simulink library "sensors_T2_lib"  (Simulink 6.6)
undefined symbols (not defined in the file or in its folder): alphavl_offset, alphavl_pos, alphavl_upwash, alphavr_offset, alphavr_pos, alphavr_upwash, betavl_offset, betavl_pos, betavl_sidewash, betavr_offset, betavr_pos, betavr_sidewash, POS_hi, POS_lo, Timestep
libraries: aeroutilslib x29, simulink_extras x6, SignalConditioning_lib x2, sensors_lib x1, simulink x1
(part 1 of 2)
settings Model: Creator=amurch  LastModifiedBy=amurch

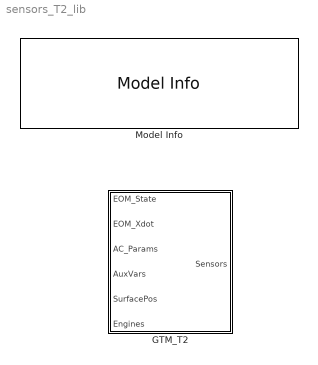
== system sensors_T2_lib ==
  GTM_T2 : Subsystem
      mask init:
      | if ~exist('MAG3TempComp','var')
      |     appendmws(Cal_params_T2)
      | end
  Model Info : simulink/Model-Wide Utilities/Model Info  SystemSampleTime=-1  InitialBlockCM=None  BlockCM=None  Frame=on  DisplayStringWithTags=|  HorizontalTextAlignment=Center  LeftAlignmentValue=0.5  SourceBlockDiagram=sensors_T2_lib  TagMaxNumber=20
      | GTM T2 Sensor Model Library
      | %<ModelVersion>
      | Las modified by %<LastModifiedBy> on %<LastModificationDate>

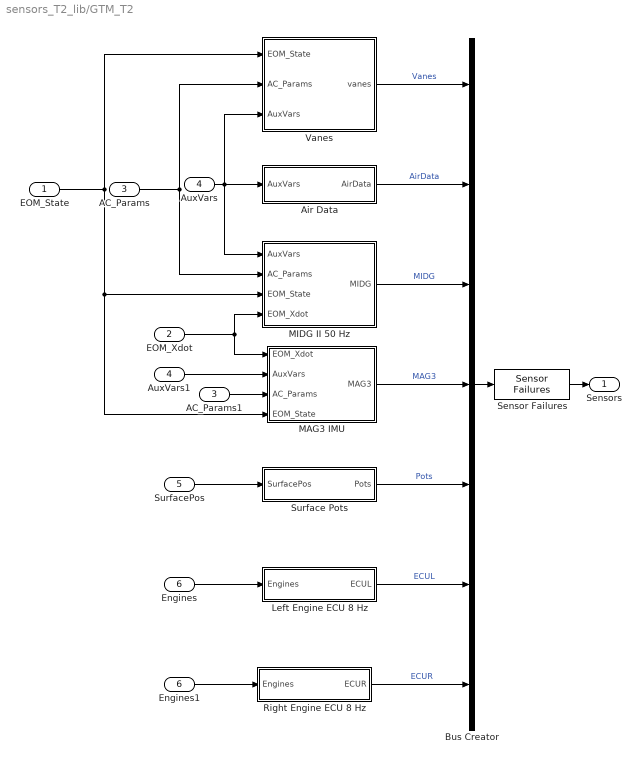
== system sensors_T2_lib/GTM_T2 ==
  EOM_State : Inport
  EOM_Xdot : Inport  Port=2
  AC_Params : Inport  Port=3
  AuxVars : Inport  Port=4
  SurfacePos : Inport  Port=5
  Engines : Inport  Port=6
  AC_Params1 : InportShadow  Port=3  LatchByCopyingInsideSignal=off
  Air Data : Subsystem
  AuxVars1 : InportShadow  Port=4  LatchByCopyingInsideSignal=off
  Bus Creator : BusCreator  Inputs=7
  Engines1 : InportShadow  Port=6  LatchByCopyingInsideSignal=off
  Left Engine ECU 8 Hz : Subsystem  SystemSampleTime=round(1/Timestep/8)*Timestep
  MAG3 IMU : Subsystem
  MIDG II 50 Hz : Subsystem  SystemSampleTime=round(1/Timestep/50)*Timestep
  Right Engine ECU 8 Hz : Subsystem  SystemSampleTime=round(1/Timestep/8)*Timestep
  Sensor Failures : sensors_lib/Sensor Failures  SystemSampleTime=-1
  Surface Pots : Subsystem
  Vanes : Subsystem
  Sensors : Outport
  wires:
  Sensor Failures/1 -> Sensors/1
  Engines1/1 -> Right Engine ECU 8 Hz/1(Engines)
  Right Engine ECU 8 Hz/1(ECUR) -> Bus Creator/7  "ECUR"
  Bus Creator/1 -> Sensor Failures/1
  Vanes/1(vanes) -> Bus Creator/1  "Vanes"
  Air Data/1(AirData) -> Bus Creator/2  "AirData"
  MIDG II 50 Hz/1(MIDG) -> Bus Creator/3  "MIDG"
  Surface Pots/1(Pots) -> Bus Creator/5  "Pots"
  Left Engine ECU 8 Hz/1(ECUL) -> Bus Creator/6  "ECUL"
  MAG3 IMU/1(MAG3) -> Bus Creator/4  "MAG3"
  Engines/1 -> Left Engine ECU 8 Hz/1(Engines)
  SurfacePos/1 -> Surface Pots/1(SurfacePos)
  AuxVars/1 -> Air Data/1(AuxVars), Vanes/3(AuxVars), MIDG II 50 Hz/1(AuxVars)
  AC_Params/1 -> Vanes/2(AC_Params), MIDG II 50 Hz/2(AC_Params)
  EOM_State/1 -> Vanes/1(EOM_State), MIDG II 50 Hz/3(EOM_State), MAG3 IMU/4(EOM_State)
  EOM_Xdot/1 -> MIDG II 50 Hz/4(EOM_Xdot), MAG3 IMU/1(EOM_Xdot)
  AuxVars1/1 -> MAG3 IMU/2(AuxVars)
  AC_Params1/1 -> MAG3 IMU/3(AC_Params)

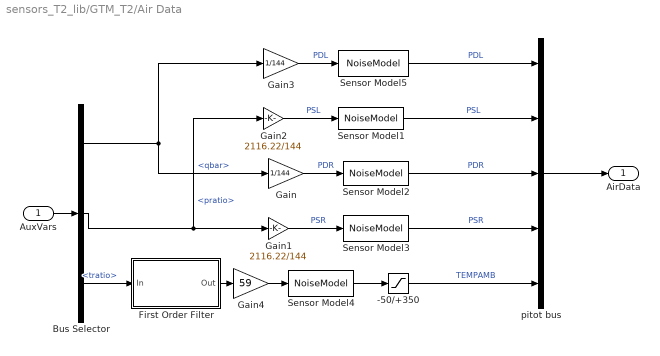
== system sensors_T2_lib/GTM_T2/Air Data ==
  AuxVars : Inport
  -50/+350 : Saturate  UpperLimit=350  LowerLimit=-50
  Bus Selector : BusSelector  OutputSignals=qbar,pratio,tratio
  First Order Filter : Subsystem  mask(first order filter){tau=6}
      mask help:
      | __1__
      |  tau s+1
      |
      | First order filter  transfer function
      | with integrator IC = input  at time=0
      | If tau < Simulation Timestep, input is passed through unchanged
      | Simulation timestep must be a variable in the model/base workspace named
      | "Timestep"
      mask Help:
      | This block models a first order filter with the initial condition
      | on the integrator set to the steady state value for constant input.
      | time constant is an input
      mask Display: fprintf('  1\n--------------\n %2.1g s + 1', tau)
  Gain : Gain  Gain=1/144
  Gain1 : Gain  Gain=2116.22/144
  Gain2 : Gain  Gain=2116.22/144
  Gain3 : Gain  Gain=1/144
  Gain4 : Gain  Gain=59
  Sensor Model1 : aeroutilslib/NoiseModel  SystemSampleTime=-1  noise_on=SensorNoise.On  sigma=SensorNoise.static_press.Std  seed=879234  bias=SensorNoise.static_press.Bias  scf=SensorNoise.static_press.Scf
  Sensor Model2 : aeroutilslib/NoiseModel  SystemSampleTime=-1  noise_on=SensorNoise.On  sigma=SensorNoise.dyn_press.Std  seed=848234  bias=SensorNoise.dyn_press.Bias  scf=SensorNoise.dyn_press.Scf
  Sensor Model3 : aeroutilslib/NoiseModel  SystemSampleTime=-1  noise_on=SensorNoise.On  sigma=SensorNoise.static_press.Std  seed=878634  bias=SensorNoise.static_press.Bias  scf=SensorNoise.static_press.Scf
  Sensor Model4 : aeroutilslib/NoiseModel  SystemSampleTime=-1  noise_on=SensorNoise.On  sigma=SensorNoise.tempamb.Std  seed=878634  bias=SensorNoise.tempamb.Bias  scf=SensorNoise.tempamb.Scf
  Sensor Model5 : aeroutilslib/NoiseModel  SystemSampleTime=-1  noise_on=SensorNoise.On  sigma=SensorNoise.dyn_press.Std  seed=878239  bias=SensorNoise.dyn_press.Bias  scf=SensorNoise.dyn_press.Scf
  pitot bus : BusCreator  Inputs=5
  AirData : Outport
  wires:
  AuxVars/1 -> Bus Selector/1
  pitot bus/1 -> AirData/1
  Bus Selector/1 -> Gain/1, Gain3/1  "<qbar>"
  Bus Selector/2 -> Gain1/1, Gain2/1  "<pratio>"
  Gain/1 -> Sensor Model2/1  "PDR"
  Gain1/1 -> Sensor Model3/1  "PSR"
  Gain3/1 -> Sensor Model5/1  "PDL"
  Gain2/1 -> Sensor Model1/1  "PSL"
  Sensor Model5/1 -> pitot bus/1  "PDL"
  Sensor Model1/1 -> pitot bus/2  "PSL"
  Sensor Model2/1 -> pitot bus/3  "PDR"
  Sensor Model3/1 -> pitot bus/4  "PSR"
  Bus Selector/3 -> First Order Filter/1(In)  "<tratio>"
  Gain4/1 -> Sensor Model4/1
  Sensor Model4/1 -> -50/+350/1
  -50/+350/1 -> pitot bus/5  "TEMPAMB"
  First Order Filter/1(Out) -> Gain4/1

== system sensors_T2_lib/GTM_T2/Left Engine ECU 8 Hz ==
  Engines : Inport
  0.025 V resolution : Quantizer  QuantizationInterval=0.025
  4.6 deg C resolution : Quantizer  QuantizationInterval=4.6
  500 RPM resolution : Quantizer  QuantizationInterval=500
  8 Hz : ZeroOrderHold  SampleTime=round(1/Timestep/8)*Timestep
  Bus Creator : BusCreator  Inputs=5
  Bus Selector : BusSelector  OutputSignals=RPML,EGTL,THROTLC,PUMPVL
  Gain : Gain
  Mode: 1 = on : Constant
  RT : RateTransition
  ECUL : Outport
  wires:
  Gain/1 -> Bus Creator/3  "ENGTL"
  Bus Selector/4 -> 0.025 V resolution/1  "<PUMPVL>"
  Bus Selector/2 -> 4.6 deg C resolution/1  "<EGTL>"
  8 Hz/1 -> RT/1
  Bus Creator/1 -> 8 Hz/1
  RT/1 -> ECUL/1
  Bus Selector/1 -> 500 RPM resolution/1  "<RPML>"
  500 RPM resolution/1 -> Bus Creator/1  "RPML"
  4.6 deg C resolution/1 -> Bus Creator/2  "EGTL"
  Bus Selector/3 -> Gain/1  "<THROTLC>"
  Mode: 1 = on/1 -> Bus Creator/5  "ENGML"
  0.025 V resolution/1 -> Bus Creator/4  "PUMPLV"
  Engines/1 -> Bus Selector/1

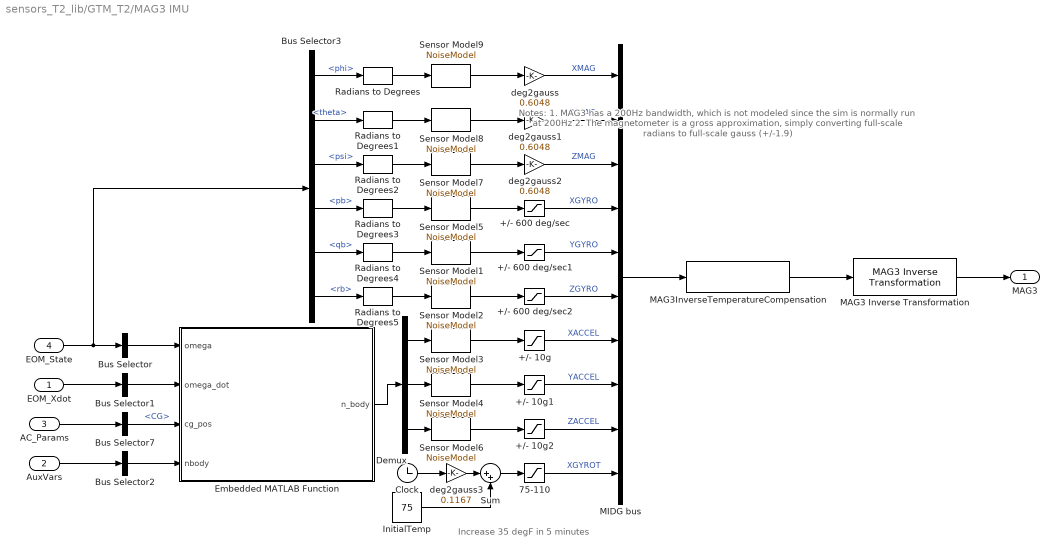
== system sensors_T2_lib/GTM_T2/MAG3 IMU ==
  note: Notes:
      |
      | 1. MAG3 has a 200Hz bandwidth, which is not modeled
      | since the sim is normally run at 200Hz
      |
      | 2.  The magnetometer is a gross approximation, simply converting
      | full-scale radians to full-scale gauss (+/-1.9)
  note: Increase 35 degF in 5 minutes
  EOM_Xdot : Inport
  AuxVars : Inport  Port=2
  AC_Params : Inport  Port=3
  EOM_State : Inport  Port=4
  +/- 10g : Saturate  UpperLimit=10  LowerLimit=-10
  +/- 10g1 : Saturate  UpperLimit=10  LowerLimit=-10
  +/- 10g2 : Saturate  UpperLimit=10  LowerLimit=-10
  +/- 600 deg/sec : Saturate  UpperLimit=600  LowerLimit=-600
  +/- 600 deg/sec1 : Saturate  UpperLimit=600  LowerLimit=-600
  +/- 600 deg/sec2 : Saturate  UpperLimit=600  LowerLimit=-600
  75-110 : Saturate  UpperLimit=110  LowerLimit=75
  Bus Selector : BusSelector  OutputSignals=pb,qb,rb  OutputAsBus=on
  Bus Selector1 : BusSelector  OutputSignals=pb_dot,qb_dot,rb_dot  OutputAsBus=on
  Bus Selector2 : BusSelector  OutputSignals=Ax,Ay,Az  OutputAsBus=on
  Bus Selector3 : BusSelector  OutputSignals=phi,theta,psi,pb,qb,rb
  Bus Selector7 : BusSelector  OutputSignals=CG
  Clock : Clock
      settings: Decimation=10
  Demux : Demux  Outputs=3
  Embedded MATLAB Function : Stateflow chart
  InitialTemp : Constant  Value=75
  MAG3 Inverse Transformation : SignalConditioning_lib/MAG3 Inverse Transformation  SystemSampleTime=-1
  MAG3InverseTemperatureCompensation : SignalConditioning_lib/MAG3InverseTemperatureCompensation  SystemSampleTime=-1
  MIDG bus : BusCreator  Inputs=10
  Radians to Degrees{,1..5} (6 alike) : simulink_extras/Transformations/Radians to Degrees  SystemSampleTime=-1
  Sensor Model1 : aeroutilslib/NoiseModel  SystemSampleTime=-1  noise_on=SensorNoise.On  sigma=SensorNoise.MAG3.qdeg.Std  seed=871234  bias=SensorNoise.MAG3.qdeg.Bias  scf=SensorNoise.MAG3.qdeg.Scf
  Sensor Model2 : aeroutilslib/NoiseModel  SystemSampleTime=-1  noise_on=SensorNoise.On  sigma=SensorNoise.MAG3.rdeg.Std  seed=878134  bias=SensorNoise.MAG3.rdeg.Bias  scf=SensorNoise.MAG3.rdeg.Scf
  Sensor Model3 : aeroutilslib/NoiseModel  SystemSampleTime=-1  noise_on=SensorNoise.On  sigma=SensorNoise.MAG3.nxbody.Std  seed=878234  bias=SensorNoise.MAG3.nxbody.Bias  scf=SensorNoise.MAG3.nxbody.Scf
  Sensor Model4 : aeroutilslib/NoiseModel  SystemSampleTime=-1  noise_on=SensorNoise.On  sigma=SensorNoise.MAG3.nybody.Std  seed=8782345  bias=SensorNoise.MAG3.nybody.Bias  scf=SensorNoise.MAG3.nybody.Scf
  Sensor Model5 : aeroutilslib/NoiseModel  SystemSampleTime=-1  noise_on=SensorNoise.On  sigma=SensorNoise.MAG3.pdeg.Std  seed=878233  bias=SensorNoise.MAG3.pdeg.Bias  scf=SensorNoise.MAG3.pdeg.Scf
  Sensor Model6 : aeroutilslib/NoiseModel  SystemSampleTime=-1  noise_on=SensorNoise.On  sigma=SensorNoise.MAG3.nzbody.Std  seed=878236  bias=SensorNoise.MAG3.nzbody.Bias  scf=SensorNoise.MAG3.nzbody.Scf
  Sensor Model7 : aeroutilslib/NoiseModel  SystemSampleTime=-1  noise_on=SensorNoise.On  sigma=SensorNoise.MAG3.psi.Std  seed=878232  bias=SensorNoise.MAG3.psi.Bias  scf=SensorNoise.MAG3.psi.Scf
  Sensor Model8 : aeroutilslib/NoiseModel  SystemSampleTime=-1  noise_on=SensorNoise.On  sigma=SensorNoise.MAG3.theta.Std  seed=878231  bias=SensorNoise.MAG3.theta.Bias  scf=SensorNoise.MAG3.theta.Scf
  Sensor Model9 : aeroutilslib/NoiseModel  SystemSampleTime=-1  noise_on=SensorNoise.On  sigma=SensorNoise.MAG3.phi.Std  seed=878230  bias=SensorNoise.MAG3.phi.Bias  scf=SensorNoise.MAG3.phi.Scf
  Sum : Sum  Inputs=|++
  deg2gauss : Gain  Gain=0.6048
  deg2gauss1 : Gain  Gain=0.6048
  deg2gauss2 : Gain  Gain=0.6048
  deg2gauss3 : Gain  Gain=0.1167
  MAG3 : Outport
  wires:
  75-110/1 -> MIDG bus/10  "XGYROT"
  Sum/1 -> 75-110/1
  deg2gauss3/1 -> Sum/1
  InitialTemp/1 -> Sum/2
  Clock/1 -> deg2gauss3/1
  MAG3 Inverse Transformation/1 -> MAG3/1
  MIDG bus/1 -> MAG3InverseTemperatureCompensation/1
  MAG3InverseTemperatureCompensation/1 -> MAG3 Inverse Transformation/1
  +/- 10g2/1 -> MIDG bus/9  "ZACCEL"
  +/- 10g1/1 -> MIDG bus/8  "YACCEL"
  +/- 10g/1 -> MIDG bus/7  "XACCEL"
  +/- 600 deg/sec2/1 -> MIDG bus/6  "ZGYRO"
  +/- 600 deg/sec1/1 -> MIDG bus/5  "YGYRO"
  +/- 600 deg/sec/1 -> MIDG bus/4  "XGYRO"
  deg2gauss2/1 -> MIDG bus/3  "ZMAG"
  deg2gauss1/1 -> MIDG bus/2  "YMAG"
  deg2gauss/1 -> MIDG bus/1  "XMAG"
  Sensor Model7/1 -> deg2gauss2/1
  Sensor Model8/1 -> deg2gauss1/1
  Sensor Model9/1 -> deg2gauss/1
  EOM_State/1 -> Bus Selector3/1, Bus Selector/1
  Embedded MATLAB Function/1(n_body) -> Demux/1
  Bus Selector/1 -> Embedded MATLAB Function/1(omega)
  EOM_Xdot/1 -> Bus Selector1/1
  Bus Selector3/1 -> Radians to Degrees/1  "<phi>"
  Bus Selector3/2 -> Radians to Degrees1/1  "<theta>"
  Bus Selector3/3 -> Radians to Degrees2/1  "<psi>"
  Bus Selector3/4 -> Radians to Degrees3/1  "<pb>"
  Bus Selector3/5 -> Radians to Degrees4/1  "<qb>"
  Bus Selector3/6 -> Radians to Degrees5/1  "<rb>"
  Demux/1 -> Sensor Model3/1
  Demux/2 -> Sensor Model4/1
  Demux/3 -> Sensor Model6/1
  Bus Selector1/1 -> Embedded MATLAB Function/2(omega_dot)
  Bus Selector7/1 -> Embedded MATLAB Function/3(cg_pos)  "<CG>"
  Radians to Degrees3/1 -> Sensor Model5/1
  Radians to Degrees4/1 -> Sensor Model1/1
  Radians to Degrees5/1 -> Sensor Model2/1
  Sensor Model1/1 -> +/- 600 deg/sec1/1
  Sensor Model2/1 -> +/- 600 deg/sec2/1
  Sensor Model3/1 -> +/- 10g/1
  Sensor Model4/1 -> +/- 10g1/1
  Sensor Model6/1 -> +/- 10g2/1
  Radians to Degrees/1 -> Sensor Model9/1
  Radians to Degrees1/1 -> Sensor Model8/1
  Radians to Degrees2/1 -> Sensor Model7/1
  Sensor Model5/1 -> +/- 600 deg/sec/1
  AC_Params/1 -> Bus Selector7/1
  AuxVars/1 -> Bus Selector2/1
  Bus Selector2/1 -> Embedded MATLAB Function/4(nbody)

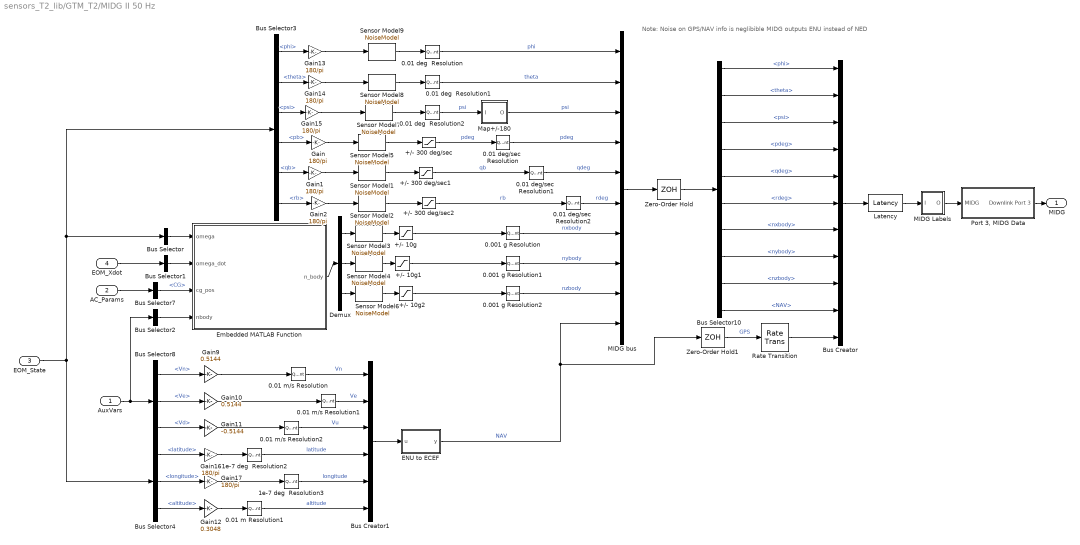
== system sensors_T2_lib/GTM_T2/MIDG II 50 Hz ==
  note: Note:  Noise on GPS/NAV info is neglibible
      | MIDG outputs ENU instead of NED
  AuxVars : Inport
  AC_Params : Inport  Port=2
  EOM_State : Inport  Port=3
  EOM_Xdot : Inport  Port=4
  +/- 10g : Saturate  UpperLimit=10  LowerLimit=-10
  +/- 10g1 : Saturate  UpperLimit=10  LowerLimit=-10
  +/- 10g2 : Saturate  UpperLimit=10  LowerLimit=-10
  +/- 300 deg/sec : Saturate  UpperLimit=300  LowerLimit=-300
  +/- 300 deg/sec1 : Saturate  UpperLimit=300  LowerLimit=-300
  +/- 300 deg/sec2 : Saturate  UpperLimit=300  LowerLimit=-300
  0.001 g Resolution : Quantizer  QuantizationInterval=0.001
  0.001 g Resolution1 : Quantizer  QuantizationInterval=0.001
  0.001 g Resolution2 : Quantizer  QuantizationInterval=0.001
  0.01 deg  Resolution : Quantizer  QuantizationInterval=0.01
  0.01 deg  Resolution1 : Quantizer  QuantizationInterval=0.01
  0.01 deg  Resolution2 : Quantizer  QuantizationInterval=0.01
  0.01 deg/sec  Resolution : Quantizer  QuantizationInterval=0.01
  0.01 deg/sec  Resolution1 : Quantizer  QuantizationInterval=0.01
  0.01 deg/sec  Resolution2 : Quantizer  QuantizationInterval=0.01
  0.01 m Resolution1 : Quantizer  QuantizationInterval=0.01
  0.01 m/s Resolution : Quantizer  QuantizationInterval=0.01
  0.01 m/s Resolution1 : Quantizer  QuantizationInterval=0.01
  0.01 m/s Resolution2 : Quantizer  QuantizationInterval=0.01
  1e-7 deg  Resolution2 : Quantizer  QuantizationInterval=1e-7
  1e-7 deg  Resolution3 : Quantizer  QuantizationInterval=1e-7
  Bus Creator : BusCreator  Inputs=11
  Bus Creator1 : BusCreator  Inputs=6
  Bus Selector : BusSelector  OutputSignals=pb,qb,rb  OutputAsBus=on
  Bus Selector1 : BusSelector  OutputSignals=pb_dot,qb_dot,rb_dot  OutputAsBus=on
  Bus Selector10 : BusSelector  OutputSignals=phi,theta,psi,pdeg,qdeg,rdeg,nxbody,nybody,nzbody,NAV
  Bus Selector2 : BusSelector  OutputSignals=Ax,Ay,Az  OutputAsBus=on
  Bus Selector3 : BusSelector  OutputSignals=phi,theta,psi,pb,qb,rb
  Bus Selector4 : BusSelector  OutputSignals=latitude,longitude,altitude
  Bus Selector7 : BusSelector  OutputSignals=CG
  Bus Selector8 : BusSelector  OutputSignals=Vn,Ve,Vd
  Demux : Demux  Outputs=3
  ENU to ECEF : Stateflow chart
  Embedded MATLAB Function : Stateflow chart
  Gain{,1..2,13..17} (8 alike) : Gain  Gain=180/pi
  Gain10 : Gain  Gain=0.5144
  Gain11 : Gain  Gain=-0.5144
  Gain12 : Gain  Gain=0.3048
  Gain9 : Gain  Gain=0.5144
  Latency : aeroutilslib/Latency  SystemSampleTime=-1  Latency=.04  timestep=Timestep
  MIDG Labels : Subsystem
  MIDG bus : BusCreator  Inputs=10
  Map+/-180 : Subsystem
  "Port 3, MIDG Data" : Subsystem
  Rate Transition : RateTransition  OutPortSampleTime=round(1/Timestep/50)*Timestep
  Sensor Model1 : aeroutilslib/NoiseModel  SystemSampleTime=-1  noise_on=SensorNoise.On  sigma=SensorNoise.MIDG.qdeg.Std  seed=871234  bias=SensorNoise.MIDG.qdeg.Bias  scf=SensorNoise.MIDG.qdeg.Scf
  Sensor Model2 : aeroutilslib/NoiseModel  SystemSampleTime=-1  noise_on=SensorNoise.On  sigma=SensorNoise.MIDG.rdeg.Std  seed=878134  bias=SensorNoise.MIDG.rdeg.Bias  scf=SensorNoise.MIDG.rdeg.Scf
  Sensor Model3 : aeroutilslib/NoiseModel  SystemSampleTime=-1  noise_on=SensorNoise.On  sigma=SensorNoise.MIDG.nxbody.Std  seed=878234  bias=SensorNoise.MIDG.nxbody.Bias  scf=SensorNoise.MIDG.nxbody.Scf
  Sensor Model4 : aeroutilslib/NoiseModel  SystemSampleTime=-1  noise_on=SensorNoise.On  sigma=SensorNoise.MIDG.nybody.Std  seed=8782345  bias=SensorNoise.MIDG.nybody.Bias  scf=SensorNoise.MIDG.nybody.Scf
  Sensor Model5 : aeroutilslib/NoiseModel  SystemSampleTime=-1  noise_on=SensorNoise.On  sigma=SensorNoise.MIDG.pdeg.Std  seed=878233  bias=SensorNoise.MIDG.pdeg.Bias  scf=SensorNoise.MIDG.pdeg.Scf
  Sensor Model6 : aeroutilslib/NoiseModel  SystemSampleTime=-1  noise_on=SensorNoise.On  sigma=SensorNoise.MIDG.nzbody.Std  seed=878236  bias=SensorNoise.MIDG.nzbody.Bias  scf=SensorNoise.MIDG.nzbody.Scf
  Sensor Model7 : aeroutilslib/NoiseModel  SystemSampleTime=-1  noise_on=SensorNoise.On  sigma=SensorNoise.MIDG.psi.Std  seed=878232  bias=SensorNoise.MIDG.psi.Bias  scf=SensorNoise.MIDG.psi.Scf
  Sensor Model8 : aeroutilslib/NoiseModel  SystemSampleTime=-1  noise_on=SensorNoise.On  sigma=SensorNoise.MIDG.theta.Std  seed=878231  bias=SensorNoise.MIDG.theta.Bias  scf=SensorNoise.MIDG.theta.Scf
  Sensor Model9 : aeroutilslib/NoiseModel  SystemSampleTime=-1  noise_on=SensorNoise.On  sigma=SensorNoise.MIDG.phi.Std  seed=878230  bias=SensorNoise.MIDG.phi.Bias  scf=SensorNoise.MIDG.phi.Scf
  Zero-Order Hold : ZeroOrderHold  SampleTime=round(1/Timestep/50)*Timestep
  Zero-Order Hold1 : ZeroOrderHold  SampleTime=round(1/Timestep/5)*Timestep
  MIDG : Outport
  wires:
  "Port 3, MIDG Data"/1(Downlink Port 3) -> MIDG/1
  Zero-Order Hold/1 -> Bus Selector10/1
  Rate Transition/1 -> Bus Creator/11
  Zero-Order Hold1/1 -> Rate Transition/1  "GPS"
  EOM_State/1 -> Bus Selector4/1, Bus Selector3/1, Bus Selector/1
  Embedded MATLAB Function/1(n_body) -> Demux/1
  EOM_Xdot/1 -> Bus Selector1/1
  Bus Selector3/1 -> Gain13/1  "<phi>"
  Bus Selector3/2 -> Gain14/1  "<theta>"
  Bus Selector3/3 -> Gain15/1  "<psi>"
  Bus Selector3/4 -> Gain/1  "<pb>"
  Bus Selector3/5 -> Gain1/1  "<qb>"
  Bus Selector3/6 -> Gain2/1  "<rb>"
  Demux/1 -> Sensor Model3/1
  Demux/2 -> Sensor Model4/1
  Demux/3 -> Sensor Model6/1
  Bus Selector7/1 -> Embedded MATLAB Function/3(cg_pos)  "<CG>"
  +/- 300 deg/sec/1 -> 0.01 deg/sec  Resolution/1  "pdeg"
  +/- 300 deg/sec1/1 -> 0.01 deg/sec  Resolution1/1  "qb"
  +/- 300 deg/sec2/1 -> 0.01 deg/sec  Resolution2/1  "rb"
  Gain/1 -> Sensor Model5/1
  Gain1/1 -> Sensor Model1/1
  Gain2/1 -> Sensor Model2/1
  +/- 10g/1 -> 0.001 g Resolution/1
  +/- 10g1/1 -> 0.001 g Resolution1/1
  Bus Creator1/1 -> ENU to ECEF/1(u)
  Bus Creator/1 -> Latency/1
  Sensor Model1/1 -> +/- 300 deg/sec1/1
  Sensor Model2/1 -> +/- 300 deg/sec2/1
  +/- 10g2/1 -> 0.001 g Resolution2/1
  Sensor Model3/1 -> +/- 10g/1
  Sensor Model4/1 -> +/- 10g1/1
  Sensor Model6/1 -> +/- 10g2/1
  Sensor Model7/1 -> 0.01 deg  Resolution2/1
  Sensor Model8/1 -> 0.01 deg  Resolution1/1
  Sensor Model9/1 -> 0.01 deg  Resolution/1
  0.01 deg  Resolution/1 -> MIDG bus/1  "phi"
  0.01 deg  Resolution1/1 -> MIDG bus/2  "theta"
  0.01 deg  Resolution2/1 -> Map+/-180/1(I)  "psi"
  1e-7 deg  Resolution2/1 -> Bus Creator1/4  "latitude"
  1e-7 deg  Resolution3/1 -> Bus Creator1/5  "longitude"
  0.001 g Resolution/1 -> MIDG bus/7  "nxbody"
  0.001 g Resolution1/1 -> MIDG bus/8  "nybody"
  0.001 g Resolution2/1 -> MIDG bus/9  "nzbody"
  0.01 m Resolution1/1 -> Bus Creator1/6  "altitude"
  Gain9/1 -> 0.01 m/s Resolution/1
  Gain10/1 -> 0.01 m/s Resolution1/1
  Gain11/1 -> 0.01 m/s Resolution2/1
  Gain12/1 -> 0.01 m Resolution1/1
  0.01 m/s Resolution/1 -> Bus Creator1/1  "Vn"
  0.01 m/s Resolution1/1 -> Bus Creator1/2  "Ve"
  0.01 m/s Resolution2/1 -> Bus Creator1/3  "Vu"
  0.01 deg/sec  Resolution1/1 -> MIDG bus/5  "qdeg"
  0.01 deg/sec  Resolution2/1 -> MIDG bus/6  "rdeg"
  MIDG bus/1 -> Zero-Order Hold/1
  Gain13/1 -> Sensor Model9/1
  Gain14/1 -> Sensor Model8/1
  Gain15/1 -> Sensor Model7/1
  Gain16/1 -> 1e-7 deg  Resolution2/1
  Gain17/1 -> 1e-7 deg  Resolution3/1
  AC_Params/1 -> Bus Selector7/1
  MIDG Labels/1(O) -> "Port 3, MIDG Data"/1(MIDG)
  Bus Selector10/1 -> Bus Creator/1  "<phi>"
  Bus Selector10/2 -> Bus Creator/2  "<theta>"
  Bus Selector10/3 -> Bus Creator/3  "<psi>"
  Bus Selector10/4 -> Bus Creator/4  "<pdeg>"
  Bus Selector10/5 -> Bus Creator/5  "<qdeg>"
  Bus Selector10/6 -> Bus Creator/6  "<rdeg>"
  Bus Selector10/7 -> Bus Creator/7  "<nxbody>"
  Bus Selector10/8 -> Bus Creator/8  "<nybody>"
  Bus Selector10/9 -> Bus Creator/9  "<nzbody>"
  Bus Selector10/10 -> Bus Creator/10  "<NAV>"
  Bus Selector8/1 -> Gain9/1  "<Vn>"
  Bus Selector8/2 -> Gain10/1  "<Ve>"
  Bus Selector8/3 -> Gain11/1  "<Vd>"
  Bus Selector4/1 -> Gain16/1  "<latitude>"
  Bus Selector4/2 -> Gain17/1  "<longitude>"
  Bus Selector4/3 -> Gain12/1  "<altitude>"
  ENU to ECEF/1(y) -> Zero-Order Hold1/1, MIDG bus/10  "NAV"
  AuxVars/1 -> Bus Selector8/1, Bus Selector2/1
  Sensor Model5/1 -> +/- 300 deg/sec/1
  0.01 deg/sec  Resolution/1 -> MIDG bus/4  "pdeg"
  Latency/1 -> MIDG Labels/1(I)
  Map+/-180/1(O) -> MIDG bus/3  "psi"
  Bus Selector/1 -> Embedded MATLAB Function/1(omega)
  Bus Selector1/1 -> Embedded MATLAB Function/2(omega_dot)
  Bus Selector2/1 -> Embedded MATLAB Function/4(nbody)

== system sensors_T2_lib/GTM_T2/Right Engine ECU 8 Hz ==
  Engines : Inport
  0.025 V resolution : Quantizer  QuantizationInterval=0.025
  4.6 deg C resolution : Quantizer  QuantizationInterval=4.6
  500 RPM resolution : Quantizer  QuantizationInterval=500
  8 Hz : ZeroOrderHold  SampleTime=round(1/Timestep/8)*Timestep
  Bus Creator : BusCreator  Inputs=5
  Bus Selector : BusSelector  OutputSignals=RPMR,EGTR,THROTRC,PUMPVR
  Gain : Gain
  Mode: 1 = on : Constant
  RT : RateTransition
  ECUR : Outport
  wires:
  Engines/1 -> Bus Selector/1
  0.025 V resolution/1 -> Bus Creator/4  "PUMPRV"
  Mode: 1 = on/1 -> Bus Creator/5  "ENGMR"
  Bus Selector/3 -> Gain/1  "<THROTRC>"
  4.6 deg C resolution/1 -> Bus Creator/2  "EGTR"
  500 RPM resolution/1 -> Bus Creator/1  "RPMR"
  Bus Selector/1 -> 500 RPM resolution/1  "<RPMR>"
  RT/1 -> ECUR/1
  Bus Creator/1 -> 8 Hz/1
  8 Hz/1 -> RT/1
  Bus Selector/2 -> 4.6 deg C resolution/1  "<EGTR>"
  Bus Selector/4 -> 0.025 V resolution/1  "<PUMPVR>"
  Gain/1 -> Bus Creator/3  "ENGTR"

== system sensors_T2_lib/GTM_T2/Surface Pots ==
  SurfacePos : Inport
  Bus Selector : BusSelector  OutputSignals=ELLOB,ELLIB,ELROB,ELRIB,AILL,AILR,RUDU,RUDL,FLAPLIB,FLAPLOB,FLAPRIB,FLAPROB  OutputAsBus=on
  Sensor Model5 : aeroutilslib/NoiseModel  SystemSampleTime=-1  noise_on=SensorNoise.On  sigma=SensorNoise.pots.Std  seed=878239  bias=SensorNoise.pots.Bias  scf=SensorNoise.pots.Scf
  Surface Labels : Subsystem
  Pots : Outport
  wires:
  Bus Selector/1 -> Sensor Model5/1
  SurfacePos/1 -> Bus Selector/1
  Sensor Model5/1 -> Surface Labels/1(I)
  Surface Labels/1(O) -> Pots/1

== system sensors_T2_lib/GTM_T2/Vanes ==
  EOM_State : Inport
  AC_Params : Inport  Port=2
  AuxVars : Inport  Port=3
  Bus Selector : BusSelector  OutputSignals=alpha,beta,tas
  Bus Selector1 : BusSelector  OutputSignals=pb,qb,rb  OutputAsBus=on
  Bus Selector2 : BusSelector  OutputSignals=CG
  Embedded MATLAB Function : Stateflow chart
  Sensor Model1 : aeroutilslib/NoiseModel  SystemSampleTime=-1  noise_on=SensorNoise.On  sigma=SensorNoise.beta.Std  seed=878224  bias=SensorNoise.beta.Bias  scf=SensorNoise.beta.Scf
  Sensor Model2 : aeroutilslib/NoiseModel  SystemSampleTime=-1  noise_on=SensorNoise.On  sigma=SensorNoise.alpha.Std  seed=878434  bias=SensorNoise.alpha.Bias  scf=SensorNoise.alpha.Scf
  Sensor Model3 : aeroutilslib/NoiseModel  SystemSampleTime=-1  noise_on=SensorNoise.On  sigma=SensorNoise.beta.Std  seed=878534  bias=SensorNoise.beta.Bias  scf=SensorNoise.beta.Scf
  Sensor Model5 : aeroutilslib/NoiseModel  SystemSampleTime=-1  noise_on=SensorNoise.On  sigma=SensorNoise.alpha.Std  seed=278234  bias=SensorNoise.alpha.Bias  scf=SensorNoise.alpha.Scf
  vane bus : BusCreator
  vanes : Outport
  wires:
  vane bus/1 -> vanes/1
  Embedded MATLAB Function/1(alphavl) -> Sensor Model5/1
  Embedded MATLAB Function/2(betavl) -> Sensor Model1/1
  Embedded MATLAB Function/3(alphavr) -> Sensor Model2/1
  Embedded MATLAB Function/4(betavr) -> Sensor Model3/1
  AuxVars/1 -> Bus Selector/1
  Bus Selector/1 -> Embedded MATLAB Function/2(alpha)  "<alpha>"
  Bus Selector/2 -> Embedded MATLAB Function/3(beta)  "<beta>"
  Bus Selector1/1 -> Embedded MATLAB Function/1(omega)
  EOM_State/1 -> Bus Selector1/1
  Bus Selector/3 -> Embedded MATLAB Function/4(vt)  "<tas>"
  AC_Params/1 -> Bus Selector2/1
  Bus Selector2/1 -> Embedded MATLAB Function/5(cg_pos)  "<CG>"
  Sensor Model5/1 -> vane bus/1  "ALPHAVL"
  Sensor Model1/1 -> vane bus/2  "BETAVL"
  Sensor Model2/1 -> vane bus/3  "ALPHAVR"
  Sensor Model3/1 -> vane bus/4  "BETAVR"

== system sensors_T2_lib/GTM_T2/Air Data/First Order Filter ==
  In : Inport
  Constant : Constant  Value=Timestep
  Constant1 : Constant  Value=tau
  Enabled Subsystem : Subsystem  TreatAsAtomicUnit=on
  Relational Operator : RelationalOperator  Operator=>  LogicOutDataTypeMode=Boolean
  Switch : Switch  Threshold=0.5
  Out : Outport
  wires:
  Constant1/1 -> Enabled Subsystem/2(tau), Relational Operator/1
  Enabled Subsystem/1(Out) -> Switch/1
  Switch/1 -> Out/1
  In/1 -> Enabled Subsystem/1(In), Switch/3
  Relational Operator/1 -> Enabled Subsystem/Enable, Switch/2
  Constant/1 -> Relational Operator/2

== system sensors_T2_lib/GTM_T2/MIDG II 50 Hz/MIDG Labels ==
  I : Inport
  Bus Creator : BusCreator  Inputs=33
  Demux : Demux  Outputs=33
  O : Outport
  wires:
  I/1 -> Demux/1
  Bus Creator/1 -> O/1
  Demux/2 -> Bus Creator/2  "theta"
  Demux/3 -> Bus Creator/3  "psi"
  Demux/4 -> Bus Creator/4  "pdeg"
  Demux/5 -> Bus Creator/5  "qdeg"
  Demux/6 -> Bus Creator/6  "rdeg"
  Demux/7 -> Bus Creator/7  "nxbody"
  Demux/8 -> Bus Creator/8  "nybody"
  Demux/9 -> Bus Creator/9  "nzbody"
  Demux/10 -> Bus Creator/10  "NAV_latitude"
  Demux/11 -> Bus Creator/11  "NAV_longitude"
  Demux/12 -> Bus Creator/12  "NAV_altitude"
  Demux/13 -> Bus Creator/13  "NAV_Vn"
  Demux/14 -> Bus Creator/14  "NAV_Ve"
  Demux/15 -> Bus Creator/15  "NAV_Vu"
  Demux/1 -> Bus Creator/1  "phi"
  Demux/16 -> Bus Creator/16  "NAV_XE"
  Demux/17 -> Bus Creator/17  "NAV_YE"
  Demux/18 -> Bus Creator/18  "NAV_ZE"
  Demux/19 -> Bus Creator/19  "NAV_VXE"
  Demux/20 -> Bus Creator/20  "NAV_VYE"
  Demux/21 -> Bus Creator/21  "NAV_VZE"
  Demux/22 -> Bus Creator/22  "GPS_latitude"
  Demux/23 -> Bus Creator/23  "GPS_longitude"
  Demux/24 -> Bus Creator/24  "GPS_altitude"
  Demux/25 -> Bus Creator/25  "GPS_Vn"
  Demux/26 -> Bus Creator/26  "GPS_Ve"
  Demux/27 -> Bus Creator/27  "GPS_Vu"
  Demux/28 -> Bus Creator/28  "GPS_XE"
  Demux/29 -> Bus Creator/29  "GPS_YE"
  Demux/30 -> Bus Creator/30  "GPS_ZE"
  Demux/31 -> Bus Creator/31  "GPS_VXE"
  Demux/32 -> Bus Creator/32  "GPS_VYE"
  Demux/33 -> Bus Creator/33  "GPS_VZE"

== system sensors_T2_lib/GTM_T2/MIDG II 50 Hz/Map+/-180 ==
  I : Inport
  Constant : Constant  Value=-360
  Constant1 : Constant  Value=0
  Sum : Sum  Inputs=|++
  if>180sub360 : Switch  Threshold=180
  O : Outport
  wires:
  if>180sub360/1 -> Sum/2
  Sum/1 -> O/1
  I/1 -> if>180sub360/2, Sum/1
  Constant1/1 -> if>180sub360/3
  Constant/1 -> if>180sub360/1

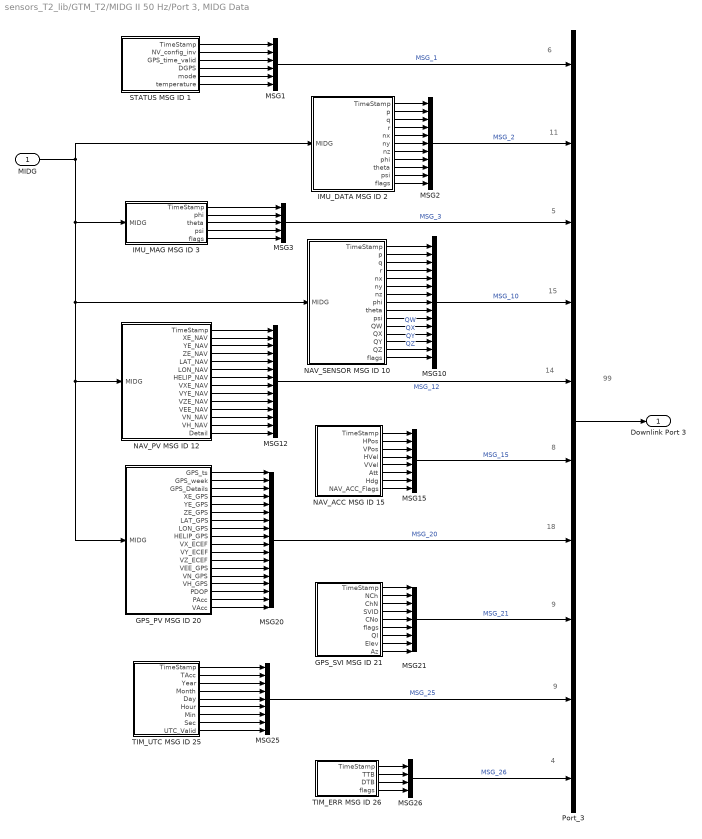
== system sensors_T2_lib/GTM_T2/MIDG II 50 Hz/Port 3, MIDG Data ==
  note: 99
  note: 4
  note: 9
  note: 9
  note: 18
  note: 8
  note: 14
  note: 15
  note: 5
  note: 11
  note: 6
  MIDG : Inport
  GPS_PV MSG ID 20 : Subsystem
  GPS_SVI MSG ID 21 : Subsystem
  IMU_DATA MSG ID 2 : Subsystem
  IMU_MAG MSG ID 3 : Subsystem
  MSG1 : BusCreator  Inputs=6
  MSG10 : BusCreator  Inputs=15
  MSG12 : BusCreator  Inputs=14
  MSG15 : BusCreator  Inputs=8
  MSG2 : BusCreator  Inputs=11
  MSG20 : BusCreator  Inputs=18
  MSG21 : BusCreator  Inputs=9
  MSG25 : BusCreator  Inputs=9
  MSG26 : BusCreator
  MSG3 : BusCreator  Inputs=5
  NAV_ACC MSG ID 15 : Subsystem
  NAV_PV MSG ID 12 : Subsystem
  NAV_SENSOR MSG ID 10 : Subsystem
  Port_3 : BusCreator  Inputs=10
  STATUS MSG ID 1 : Subsystem
  TIM_ERR MSG ID 26 : Subsystem
  TIM_UTC MSG ID 25 : Subsystem
  Downlink Port 3 : Outport
  wires:
  MIDG/1 -> IMU_DATA MSG ID 2/1(MIDG), NAV_SENSOR MSG ID 10/1(MIDG), GPS_PV MSG ID 20/1(MIDG), NAV_PV MSG ID 12/1(MIDG), IMU_MAG MSG ID 3/1(MIDG)
  Port_3/1 -> Downlink Port 3/1
  MSG21/1 -> Port_3/8  "MSG_21"
  MSG20/1 -> Port_3/7  "MSG_20"
  GPS_PV MSG ID 20/1(GPS_ts) -> MSG20/1
  GPS_PV MSG ID 20/2(GPS_week) -> MSG20/2
  GPS_PV MSG ID 20/3(GPS_Details) -> MSG20/3
  MSG10/1 -> Port_3/4  "MSG_10"
  MSG26/1 -> Port_3/10  "MSG_26"
  MSG25/1 -> Port_3/9  "MSG_25"
  MSG15/1 -> Port_3/6  "MSG_15"
  MSG12/1 -> Port_3/5  "MSG_12"
  MSG3/1 -> Port_3/3  "MSG_3"
  MSG2/1 -> Port_3/2  "MSG_2"
  MSG1/1 -> Port_3/1  "MSG_1"
  NAV_SENSOR MSG ID 10/15(flags) -> MSG10/15
  NAV_SENSOR MSG ID 10/14(QZ) -> MSG10/14  "QZ"
  NAV_SENSOR MSG ID 10/13(QY) -> MSG10/13  "QY"
  NAV_SENSOR MSG ID 10/12(QX) -> MSG10/12  "QX"
  NAV_SENSOR MSG ID 10/11(QW) -> MSG10/11  "QW"
  TIM_ERR MSG ID 26/4(flags) -> MSG26/4
  TIM_ERR MSG ID 26/3(DTB) -> MSG26/3
  TIM_ERR MSG ID 26/2(TTB) -> MSG26/2
  TIM_ERR MSG ID 26/1(TimeStamp) -> MSG26/1
  TIM_UTC MSG ID 25/9(UTC_Valid) -> MSG25/9
  TIM_UTC MSG ID 25/8(Sec) -> MSG25/8
  TIM_UTC MSG ID 25/7(Min) -> MSG25/7
  TIM_UTC MSG ID 25/6(Hour) -> MSG25/6
  TIM_UTC MSG ID 25/5(Day) -> MSG25/5
  TIM_UTC MSG ID 25/4(Month) -> MSG25/4
  TIM_UTC MSG ID 25/3(Year) -> MSG25/3
  TIM_UTC MSG ID 25/2(TAcc) -> MSG25/2
  TIM_UTC MSG ID 25/1(TimeStamp) -> MSG25/1
  GPS_SVI MSG ID 21/9(Az) -> MSG21/9
  GPS_SVI MSG ID 21/8(Elev) -> MSG21/8
  GPS_SVI MSG ID 21/7(QI) -> MSG21/7
  GPS_SVI MSG ID 21/6(flags) -> MSG21/6
  GPS_SVI MSG ID 21/5(CNo) -> MSG21/5
  GPS_SVI MSG ID 21/4(SVID) -> MSG21/4
  GPS_SVI MSG ID 21/3(ChN) -> MSG21/3
  GPS_SVI MSG ID 21/2(NCh) -> MSG21/2
  GPS_SVI MSG ID 21/1(TimeStamp) -> MSG21/1
  NAV_ACC MSG ID 15/8(NAV_ACC_Flags) -> MSG15/8
  NAV_ACC MSG ID 15/7(Hdg) -> MSG15/7
  NAV_ACC MSG ID 15/6(Att) -> MSG15/6
  NAV_ACC MSG ID 15/5(VVel) -> MSG15/5
  NAV_ACC MSG ID 15/4(HVel) -> MSG15/4
  NAV_ACC MSG ID 15/3(VPos) -> MSG15/3
  NAV_ACC MSG ID 15/2(HPos) -> MSG15/2
  NAV_ACC MSG ID 15/1(TimeStamp) -> MSG15/1
  NAV_SENSOR MSG ID 10/10(psi) -> MSG10/10
  NAV_SENSOR MSG ID 10/9(theta) -> MSG10/9
  NAV_SENSOR MSG ID 10/8(phi) -> MSG10/8
  NAV_SENSOR MSG ID 10/7(nz) -> MSG10/7
  NAV_SENSOR MSG ID 10/6(ny) -> MSG10/6
  NAV_SENSOR MSG ID 10/5(nx) -> MSG10/5
  NAV_SENSOR MSG ID 10/4(r) -> MSG10/4
  NAV_SENSOR MSG ID 10/3(q) -> MSG10/3
  NAV_SENSOR MSG ID 10/2(p) -> MSG10/2
  NAV_SENSOR MSG ID 10/1(TimeStamp) -> MSG10/1
  GPS_PV MSG ID 20/18(VAcc) -> MSG20/18
  GPS_PV MSG ID 20/17(PAcc) -> MSG20/17
  GPS_PV MSG ID 20/16(PDOP) -> MSG20/16
  GPS_PV MSG ID 20/15(VH_GPS) -> MSG20/15
  GPS_PV MSG ID 20/14(VN_GPS) -> MSG20/14
  GPS_PV MSG ID 20/13(VEE_GPS) -> MSG20/13
  GPS_PV MSG ID 20/12(VZ_ECEF) -> MSG20/12
  GPS_PV MSG ID 20/11(VY_ECEF) -> MSG20/11
  GPS_PV MSG ID 20/10(VX_ECEF) -> MSG20/10
  GPS_PV MSG ID 20/9(HELIP_GPS) -> MSG20/9
  GPS_PV MSG ID 20/8(LON_GPS) -> MSG20/8
  GPS_PV MSG ID 20/7(LAT_GPS) -> MSG20/7
  GPS_PV MSG ID 20/6(ZE_GPS) -> MSG20/6
  GPS_PV MSG ID 20/5(YE_GPS) -> MSG20/5
  GPS_PV MSG ID 20/4(XE_GPS) -> MSG20/4
  NAV_PV MSG ID 12/1(TimeStamp) -> MSG12/1
  NAV_PV MSG ID 12/2(XE_NAV) -> MSG12/2
  NAV_PV MSG ID 12/3(YE_NAV) -> MSG12/3
  NAV_PV MSG ID 12/4(ZE_NAV) -> MSG12/4
  NAV_PV MSG ID 12/5(LAT_NAV) -> MSG12/5
  NAV_PV MSG ID 12/6(LON_NAV) -> MSG12/6
  NAV_PV MSG ID 12/7(HELIP_NAV) -> MSG12/7
  NAV_PV MSG ID 12/8(VXE_NAV) -> MSG12/8
  NAV_PV MSG ID 12/9(VYE_NAV) -> MSG12/9
  NAV_PV MSG ID 12/10(VZE_NAV) -> MSG12/10
  NAV_PV MSG ID 12/11(VEE_NAV) -> MSG12/11
  NAV_PV MSG ID 12/12(VN_NAV) -> MSG12/12
  NAV_PV MSG ID 12/13(VH_NAV) -> MSG12/13
  NAV_PV MSG ID 12/14(Detail) -> MSG12/14
  IMU_MAG MSG ID 3/5(flags) -> MSG3/5
  IMU_MAG MSG ID 3/4(psi) -> MSG3/4
  IMU_MAG MSG ID 3/3(theta) -> MSG3/3
  IMU_MAG MSG ID 3/2(phi) -> MSG3/2
  IMU_MAG MSG ID 3/1(TimeStamp) -> MSG3/1
  IMU_DATA MSG ID 2/11(flags) -> MSG2/11
  IMU_DATA MSG ID 2/10(psi) -> MSG2/10
  IMU_DATA MSG ID 2/9(theta) -> MSG2/9
  IMU_DATA MSG ID 2/8(phi) -> MSG2/8
  IMU_DATA MSG ID 2/7(nz) -> MSG2/7
  IMU_DATA MSG ID 2/5(nx) -> MSG2/5
  IMU_DATA MSG ID 2/4(r) -> MSG2/4
  IMU_DATA MSG ID 2/3(q) -> MSG2/3
  IMU_DATA MSG ID 2/2(p) -> MSG2/2
  IMU_DATA MSG ID 2/1(TimeStamp) -> MSG2/1
  IMU_DATA MSG ID 2/6(ny) -> MSG2/6
  STATUS MSG ID 1/6(temperature) -> MSG1/6
  STATUS MSG ID 1/5(mode) -> MSG1/5
  STATUS MSG ID 1/4(DGPS) -> MSG1/4
  STATUS MSG ID 1/3(GPS_time_valid) -> MSG1/3
  STATUS MSG ID 1/2(NV_config_inv) -> MSG1/2
  STATUS MSG ID 1/1(TimeStamp) -> MSG1/1

== system sensors_T2_lib/GTM_T2/Surface Pots/Surface Labels ==
  I : Inport
  Bus Creator : BusCreator  Inputs=12
  Demux : Demux  Outputs=12
  O : Outport
  wires:
  Bus Creator/1 -> O/1
  Demux/12 -> Bus Creator/12  "FLAPROB"
  Demux/11 -> Bus Creator/11  "FLAPRIB"
  Demux/10 -> Bus Creator/10  "FLAPLOB"
  Demux/9 -> Bus Creator/9  "FLAPLIB"
  Demux/8 -> Bus Creator/8  "RUDL"
  Demux/7 -> Bus Creator/7  "RUDU"
  Demux/6 -> Bus Creator/6  "AILR"
  Demux/5 -> Bus Creator/5  "AILL"
  Demux/4 -> Bus Creator/4  "ELRIB"
  Demux/3 -> Bus Creator/3  "ELROB"
  Demux/2 -> Bus Creator/2  "ELLIB"
  Demux/1 -> Bus Creator/1  "ELLOB"
  I/1 -> Demux/1

== system sensors_T2_lib/GTM_T2/Air Data/First Order Filter/Enabled Subsystem ==
  In : Inport
  tau : Inport  Port=2
  Enable : EnablePort
  Divide : Product  Inputs=*/  OutScaling=2^-10
  Integrator : Integrator  InitialConditionSource=external  UpperSaturationLimit=POS_hi  LowerSaturationLimit=POS_lo
  Sum : Sum  Inputs=-+|  SaturateOnIntegerOverflow=on  InputSameDT=on
  Out : Outport
  wires:
  Sum/1 -> Divide/1  "Error"
  In/1 -> Sum/2, Integrator/2
  Integrator/1 -> Out/1, Sum/1  "Y"
  tau/1 -> Divide/2
  Divide/1 -> Integrator/1  "Ydot"

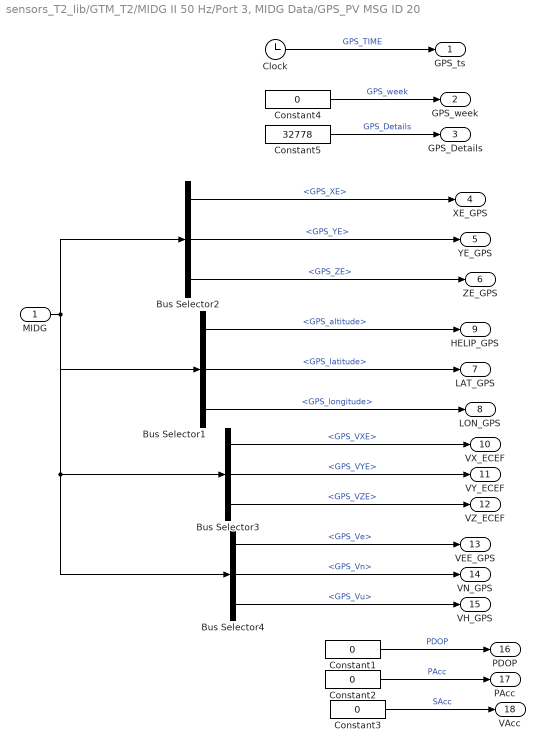
== system sensors_T2_lib/GTM_T2/MIDG II 50 Hz/Port 3, MIDG Data/GPS_PV MSG ID 20 ==
  MIDG : Inport
  Bus Selector1 : BusSelector  OutputSignals=GPS_altitude,GPS_latitude,GPS_longitude
  Bus Selector2 : BusSelector  OutputSignals=GPS_XE,GPS_YE,GPS_ZE
  Bus Selector3 : BusSelector  OutputSignals=GPS_VXE,GPS_VYE,GPS_VZE
  Bus Selector4 : BusSelector  OutputSignals=GPS_Ve,GPS_Vn,GPS_Vu
  Clock : Clock
      settings: Decimation=10
  Constant{1..4} (4 alike) : Constant  Value=0
  Constant5 : Constant  Value=32778
  GPS_ts : Outport
  GPS_week : Outport  Port=2
  GPS_Details : Outport  Port=3
  XE_GPS : Outport  Port=4
  YE_GPS : Outport  Port=5
  ZE_GPS : Outport  Port=6
  LAT_GPS : Outport  Port=7
  LON_GPS : Outport  Port=8
  HELIP_GPS : Outport  Port=9
  VX_ECEF : Outport  Port=10
  VY_ECEF : Outport  Port=11
  VZ_ECEF : Outport  Port=12
  VEE_GPS : Outport  Port=13
  VN_GPS : Outport  Port=14
  VH_GPS : Outport  Port=15
  PDOP : Outport  Port=16
  PAcc : Outport  Port=17
  VAcc : Outport  Port=18
  wires:
  Bus Selector2/3 -> ZE_GPS/1  "<GPS_ZE>"
  Bus Selector2/2 -> YE_GPS/1  "<GPS_YE>"
  Bus Selector2/1 -> XE_GPS/1  "<GPS_XE>"
  Bus Selector3/3 -> VZ_ECEF/1  "<GPS_VZE>"
  Bus Selector3/2 -> VY_ECEF/1  "<GPS_VYE>"
  Bus Selector3/1 -> VX_ECEF/1  "<GPS_VXE>"
  Constant5/1 -> GPS_Details/1  "GPS_Details"
  Constant4/1 -> GPS_week/1  "GPS_week"
  Clock/1 -> GPS_ts/1  "GPS_TIME"
  Constant3/1 -> VAcc/1  "SAcc"
  Constant2/1 -> PAcc/1  "PAcc"
  Constant1/1 -> PDOP/1  "PDOP"
  Bus Selector4/3 -> VH_GPS/1  "<GPS_Vu>"
  Bus Selector4/2 -> VN_GPS/1  "<GPS_Vn>"
  Bus Selector4/1 -> VEE_GPS/1  "<GPS_Ve>"
  Bus Selector1/3 -> LON_GPS/1  "<GPS_longitude>"
  Bus Selector1/2 -> LAT_GPS/1  "<GPS_latitude>"
  Bus Selector1/1 -> HELIP_GPS/1  "<GPS_altitude>"
  MIDG/1 -> Bus Selector2/1, Bus Selector4/1, Bus Selector3/1, Bus Selector1/1

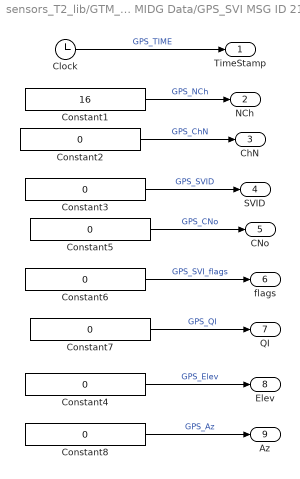
== system sensors_T2_lib/GTM_T2/MIDG II 50 Hz/Port 3, MIDG Data/GPS_SVI MSG ID 21 ==
  Clock : Clock
      settings: Decimation=10
  Constant1 : Constant  Value=16
  Constant{2..8} (7 alike) : Constant  Value=0
  TimeStamp : Outport
  NCh : Outport  Port=2
  ChN : Outport  Port=3
  SVID : Outport  Port=4
  CNo : Outport  Port=5
  flags : Outport  Port=6
  QI : Outport  Port=7
  Elev : Outport  Port=8
  Az : Outport  Port=9
  wires:
  Constant8/1 -> Az/1  "GPS_Az"
  Constant7/1 -> QI/1  "GPS_QI"
  Constant6/1 -> flags/1  "GPS_SVI_flags"
  Constant5/1 -> CNo/1  "GPS_CNo"
  Constant3/1 -> SVID/1  "GPS_SVID"
  Constant2/1 -> ChN/1  "GPS_ChN"
  Constant1/1 -> NCh/1  "GPS_NCh"
  Constant4/1 -> Elev/1  "GPS_Elev"
  Clock/1 -> TimeStamp/1  "GPS_TIME"

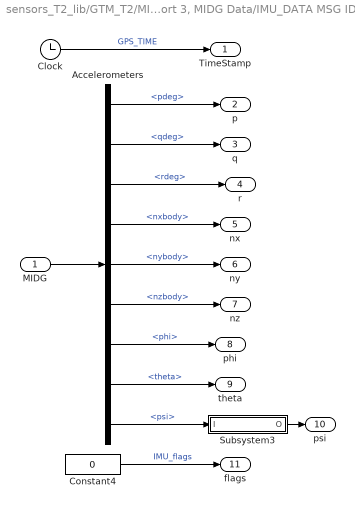
== system sensors_T2_lib/GTM_T2/MIDG II 50 Hz/Port 3, MIDG Data/IMU_DATA MSG ID 2 ==
  MIDG : Inport
  Accelerometers : BusSelector  OutputSignals=pdeg,qdeg,rdeg,nxbody,nybody,nzbody,phi,theta,psi
  Clock : Clock
      settings: Decimation=10
  Constant4 : Constant  Value=0
  Subsystem3 : Subsystem
      mask Display: disp('no windup 180')
  TimeStamp : Outport
  p : Outport  Port=2
  q : Outport  Port=3
  r : Outport  Port=4
  nx : Outport  Port=5
  ny : Outport  Port=6
  nz : Outport  Port=7
  phi : Outport  Port=8
  theta : Outport  Port=9
  psi : Outport  Port=10
  flags : Outport  Port=11
  wires:
  Accelerometers/9 -> Subsystem3/1(I)  "<psi>"
  Accelerometers/8 -> theta/1  "<theta>"
  Accelerometers/7 -> phi/1  "<phi>"
  Accelerometers/3 -> r/1  "<rdeg>"
  Accelerometers/2 -> q/1  "<qdeg>"
  Accelerometers/1 -> p/1  "<pdeg>"
  Subsystem3/1(O) -> psi/1
  Constant4/1 -> flags/1  "IMU_flags"
  Clock/1 -> TimeStamp/1  "GPS_TIME"
  Accelerometers/4 -> nx/1  "<nxbody>"
  Accelerometers/5 -> ny/1  "<nybody>"
  Accelerometers/6 -> nz/1  "<nzbody>"
  MIDG/1 -> Accelerometers/1

== system sensors_T2_lib/GTM_T2/MIDG II 50 Hz/Port 3, MIDG Data/IMU_MAG MSG ID 3 ==
  MIDG : Inport
  Clock : Clock
      settings: Decimation=10
  Constant4 : Constant  Value=0
  Magnetometer : BusSelector  OutputSignals=phi,theta,psi
  Subsystem3 : Subsystem
      mask Display: disp('no windup 180')
  TimeStamp : Outport
  phi : Outport  Port=2
  theta : Outport  Port=3
  psi : Outport  Port=4
  flags : Outport  Port=5
  wires:
  Subsystem3/1(O) -> psi/1
  Constant4/1 -> flags/1  "MAG_flags"
  Clock/1 -> TimeStamp/1  "GPS_TIME"
  Magnetometer/1 -> phi/1  "<phi>"
  Magnetometer/2 -> theta/1  "<theta>"
  Magnetometer/3 -> Subsystem3/1(I)  "<psi>"
  MIDG/1 -> Magnetometer/1

== system sensors_T2_lib/GTM_T2/MIDG II 50 Hz/Port 3, MIDG Data/NAV_ACC MSG ID 15 ==
  Clock : Clock
      settings: Decimation=10
  Constant{1..7} (7 alike) : Constant  Value=0
  TimeStamp : Outport
  HPos : Outport  Port=2
  VPos : Outport  Port=3
  HVel : Outport  Port=4
  VVel : Outport  Port=5
  Att : Outport  Port=6
  Hdg : Outport  Port=7
  NAV_ACC_Flags : Outport  Port=8
  wires:
  Constant7/1 -> Hdg/1  "Hdg"
  Constant6/1 -> Att/1  "Att"
  Constant5/1 -> VVel/1  "VVel"
  Constant3/1 -> HVel/1  "HVel"
  Constant2/1 -> VPos/1  "VPos"
  Constant1/1 -> HPos/1  "HPos"
  Constant4/1 -> NAV_ACC_Flags/1  "NAV_ACC_Flags"
  Clock/1 -> TimeStamp/1  "GPS_TIME"

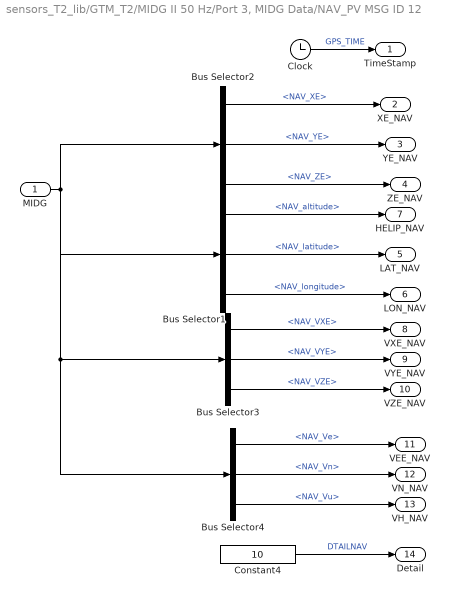
== system sensors_T2_lib/GTM_T2/MIDG II 50 Hz/Port 3, MIDG Data/NAV_PV MSG ID 12 ==
  MIDG : Inport
  Bus Selector1 : BusSelector  OutputSignals=NAV_altitude,NAV_latitude,NAV_longitude
  Bus Selector2 : BusSelector  OutputSignals=NAV_XE,NAV_YE,NAV_ZE
  Bus Selector3 : BusSelector  OutputSignals=NAV_VXE,NAV_VYE,NAV_VZE
  Bus Selector4 : BusSelector  OutputSignals=NAV_Ve,NAV_Vn,NAV_Vu
  Clock : Clock
      settings: Decimation=10
  Constant4 : Constant  Value=10
  TimeStamp : Outport
  XE_NAV : Outport  Port=2
  YE_NAV : Outport  Port=3
  ZE_NAV : Outport  Port=4
  LAT_NAV : Outport  Port=5
  LON_NAV : Outport  Port=6
  HELIP_NAV : Outport  Port=7
  VXE_NAV : Outport  Port=8
  VYE_NAV : Outport  Port=9
  VZE_NAV : Outport  Port=10
  VEE_NAV : Outport  Port=11
  VN_NAV : Outport  Port=12
  VH_NAV : Outport  Port=13
  Detail : Outport  Port=14
  wires:
  Bus Selector2/3 -> ZE_NAV/1  "<NAV_ZE>"
  Bus Selector2/2 -> YE_NAV/1  "<NAV_YE>"
  Bus Selector2/1 -> XE_NAV/1  "<NAV_XE>"
  Bus Selector3/3 -> VZE_NAV/1  "<NAV_VZE>"
  Bus Selector3/2 -> VYE_NAV/1  "<NAV_VYE>"
  Bus Selector3/1 -> VXE_NAV/1  "<NAV_VXE>"
  Constant4/1 -> Detail/1  "DTAILNAV"
  Clock/1 -> TimeStamp/1  "GPS_TIME"
  Bus Selector4/3 -> VH_NAV/1  "<NAV_Vu>"
  Bus Selector4/2 -> VN_NAV/1  "<NAV_Vn>"
  Bus Selector4/1 -> VEE_NAV/1  "<NAV_Ve>"
  Bus Selector1/3 -> LON_NAV/1  "<NAV_longitude>"
  Bus Selector1/2 -> LAT_NAV/1  "<NAV_latitude>"
  Bus Selector1/1 -> HELIP_NAV/1  "<NAV_altitude>"
  MIDG/1 -> Bus Selector2/1, Bus Selector4/1, Bus Selector3/1, Bus Selector1/1

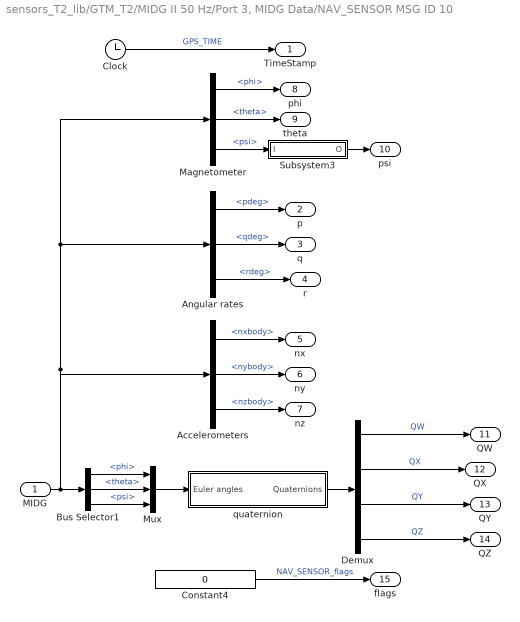
== system sensors_T2_lib/GTM_T2/MIDG II 50 Hz/Port 3, MIDG Data/NAV_SENSOR MSG ID 10 ==
  MIDG : Inport
  Accelerometers : BusSelector  OutputSignals=nxbody,nybody,nzbody
  Angular rates : BusSelector  OutputSignals=pdeg,qdeg,rdeg
  Bus Selector1 : BusSelector  OutputSignals=phi,theta,psi
  Clock : Clock
      settings: Decimation=10
  Constant4 : Constant  Value=0
  Demux : Demux
  Magnetometer : BusSelector  OutputSignals=phi,theta,psi
  Mux : Mux  Inputs=3
  Subsystem3 : Subsystem
      mask Display: disp('360 to +/-180')
  quaternion : Subsystem
  TimeStamp : Outport
  p : Outport  Port=2
  q : Outport  Port=3
  r : Outport  Port=4
  nx : Outport  Port=5
  ny : Outport  Port=6
  nz : Outport  Port=7
  phi : Outport  Port=8
  theta : Outport  Port=9
  psi : Outport  Port=10
  QW : Outport  Port=11
  QX : Outport  Port=12
  QY : Outport  Port=13
  QZ : Outport  Port=14
  flags : Outport  Port=15
  wires:
  Subsystem3/1(O) -> psi/1
  Constant4/1 -> flags/1  "NAV_SENSOR_flags"
  Clock/1 -> TimeStamp/1  "GPS_TIME"
  Angular rates/1 -> p/1  "<pdeg>"
  Angular rates/2 -> q/1  "<qdeg>"
  Angular rates/3 -> r/1  "<rdeg>"
  Accelerometers/1 -> nx/1  "<nxbody>"
  Accelerometers/2 -> ny/1  "<nybody>"
  Accelerometers/3 -> nz/1  "<nzbody>"
  Magnetometer/1 -> phi/1  "<phi>"
  Magnetometer/2 -> theta/1  "<theta>"
  Magnetometer/3 -> Subsystem3/1(I)  "<psi>"
  Bus Selector1/1 -> Mux/1  "<phi>"
  Bus Selector1/2 -> Mux/2  "<theta>"
  Bus Selector1/3 -> Mux/3  "<psi>"
  Mux/1 -> quaternion/1(Euler angles)
  quaternion/1(Quaternions) -> Demux/1
  MIDG/1 -> Accelerometers/1, Magnetometer/1, Angular rates/1, Bus Selector1/1
  Demux/1 -> QW/1  "QW"
  Demux/2 -> QX/1  "QX"
  Demux/3 -> QY/1  "QY"
  Demux/4 -> QZ/1  "QZ"

== system sensors_T2_lib/GTM_T2/MIDG II 50 Hz/Port 3, MIDG Data/STATUS MSG ID 1 ==
  note: Current Mode
      | IMU: Inertial Measuring Unit
      | VG:  Vertical Gyro
      | INS: Inertial Navigation System
      |
      | 1=IMU
      | 2=VG INIT
      | 3=VG FAST
      | 4=VG MEDIUM
      | 5=VG SLOW
      | 6=VG SE
      | 7=INS
  Clock : Clock
      settings: Decimation=10
  Constant{,1..2,4} (4 alike) : Constant  Value=0
  Constant3 : Constant  Value=7
  TimeStamp : Outport
  NV_config_inv : Outport  Port=2
  GPS_time_valid : Outport  Port=3
  DGPS : Outport  Port=4
  mode : Outport  Port=5
  temperature : Outport  Port=6
  wires:
  Constant4/1 -> temperature/1  "int_temperature"
  Constant3/1 -> mode/1  "MIDG_mode"
  Constant2/1 -> DGPS/1  "DGPS"
  Constant1/1 -> GPS_time_valid/1  "GPS_time_valid"
  Constant/1 -> NV_config_inv/1  "NV_config_inv"
  Clock/1 -> TimeStamp/1  "GPS_TIME"

== system sensors_T2_lib/GTM_T2/MIDG II 50 Hz/Port 3, MIDG Data/TIM_ERR MSG ID 26 ==
  Clock : Clock
      settings: Decimation=10
  Constant1 : Constant  Value=0
  Constant2 : Constant  Value=0
  Constant3 : Constant  Value=0
  TimeStamp : Outport
  TTB : Outport  Port=2
  DTB : Outport  Port=3
  flags : Outport  Port=4
  wires:
  Constant3/1 -> flags/1  "GPS_TimErr_flags"
  Constant2/1 -> DTB/1  "GPS_DTB"
  Constant1/1 -> TTB/1  "GPS_TTB"
  Clock/1 -> TimeStamp/1  "GPS_TIME"

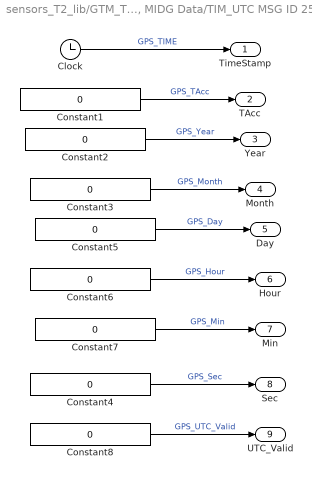
== system sensors_T2_lib/GTM_T2/MIDG II 50 Hz/Port 3, MIDG Data/TIM_UTC MSG ID 25 ==
  Clock : Clock
      settings: Decimation=10
  Constant{1..8} (8 alike) : Constant  Value=0
  TimeStamp : Outport
  TAcc : Outport  Port=2
  Year : Outport  Port=3
  Month : Outport  Port=4
  Day : Outport  Port=5
  Hour : Outport  Port=6
  Min : Outport  Port=7
  Sec : Outport  Port=8
  UTC_Valid : Outport  Port=9
  wires:
  Constant8/1 -> UTC_Valid/1  "GPS_UTC_Valid"
  Constant7/1 -> Min/1  "GPS_Min"
  Constant6/1 -> Hour/1  "GPS_Hour"
  Constant5/1 -> Day/1  "GPS_Day"
  Constant3/1 -> Month/1  "GPS_Month"
  Constant2/1 -> Year/1  "GPS_Year"
  Constant1/1 -> TAcc/1  "GPS_TAcc"
  Constant4/1 -> Sec/1  "GPS_Sec"
  Clock/1 -> TimeStamp/1  "GPS_TIME"

== system sensors_T2_lib/GTM_T2/MIDG II 50 Hz/Port 3, MIDG Data/IMU_DATA MSG ID 2/Subsystem3 ==
  I : Inport
  Constant1 : Constant  Value=2*pi
  Constant2 : Constant  Value=2*pi
  Constant3 : Constant  Value=2*pi
  Math Function1 : Math  Operator=rem  SaturateOnIntegerOverflow=on
  Sum : Sum  Inputs=|-+  SaturateOnIntegerOverflow=on
  Sum1 : Sum  Inputs=++|  SaturateOnIntegerOverflow=on
  Switch : Switch  Criteria=u2 > Threshold  Threshold=pi  SaturateOnIntegerOverflow=on
  Switch1 : Switch  SaturateOnIntegerOverflow=on
  Switch2 : Switch  Threshold=-pi  SaturateOnIntegerOverflow=on
  O : Outport
  wires:
  Constant1/1 -> Math Function1/2
  I/1 -> Math Function1/1
  Math Function1/1 -> Switch/2, Sum/2, Switch/3, Switch2/1, Switch2/2, Sum1/1, Switch1/2
  Constant2/1 -> Sum/1
  Sum/1 -> Switch/1
  Constant3/1 -> Sum1/2
  Sum1/1 -> Switch2/3
  Switch2/1 -> Switch1/3
  Switch/1 -> Switch1/1
  Switch1/1 -> O/1

== system sensors_T2_lib/GTM_T2/MIDG II 50 Hz/Port 3, MIDG Data/IMU_MAG MSG ID 3/Subsystem3 ==
  I : Inport
  Constant1 : Constant  Value=2*pi
  Constant2 : Constant  Value=2*pi
  Constant3 : Constant  Value=2*pi
  Math Function1 : Math  Operator=rem  SaturateOnIntegerOverflow=on
  Sum : Sum  Inputs=|-+  SaturateOnIntegerOverflow=on
  Sum1 : Sum  Inputs=++|  SaturateOnIntegerOverflow=on
  Switch : Switch  Criteria=u2 > Threshold  Threshold=pi  SaturateOnIntegerOverflow=on
  Switch1 : Switch  SaturateOnIntegerOverflow=on
  Switch2 : Switch  Threshold=-pi  SaturateOnIntegerOverflow=on
  O : Outport
  wires:
  Constant1/1 -> Math Function1/2
  I/1 -> Math Function1/1
  Math Function1/1 -> Switch/2, Sum/2, Switch/3, Switch2/1, Switch2/2, Sum1/1, Switch1/2
  Constant2/1 -> Sum/1
  Sum/1 -> Switch/1
  Constant3/1 -> Sum1/2
  Sum1/1 -> Switch2/3
  Switch2/1 -> Switch1/3
  Switch/1 -> Switch1/1
  Switch1/1 -> O/1

== system sensors_T2_lib/GTM_T2/MIDG II 50 Hz/Port 3, MIDG Data/NAV_SENSOR MSG ID 10/Subsystem3 ==
  I : Inport
  Constant : Constant  Value=0
  Constant4 : Constant  Value=360
  Sum2 : Sum  Inputs=|+-  SaturateOnIntegerOverflow=on
  Switch3 : Switch  Threshold=180  SaturateOnIntegerOverflow=on
  O : Outport
  wires:
  I/1 -> Switch3/2, Sum2/1
  Sum2/1 -> O/1
  Switch3/1 -> Sum2/2
  Constant/1 -> Switch3/3
  Constant4/1 -> Switch3/1

== system sensors_T2_lib/GTM_T2/MIDG II 50 Hz/Port 3, MIDG Data/NAV_SENSOR MSG ID 10/quaternion ==
  Euler angles : Inport
  1/2 : Gain  Gain=1/2  SaturateOnIntegerOverflow=on
  Cos(Euler/2) : Trigonometry  Operator=cos
  Mux1 : Mux  Inputs=2
  Mux2 : Mux
  Sin(Euler/2) : Trigonometry
  e0 : Fcn  Expr=u(1)*u(2)*u(3)+u(4)*u(5)*u(6)
  e1 : Fcn  Expr=-u(2)*u(3)*u(4)+u(1)*u(5)*u(6)
  e2 : Fcn  Expr=u(1)*u(5)*u(3)+u(2)*u(4)*u(6)
  e3 : Fcn  Expr=u(3)*u(4)*u(5)-u(1)*u(2)*u(6)
  Quaternions : Outport
  wires:
  1/2/1 -> Sin(Euler/2)/1, Cos(Euler/2)/1
  Sin(Euler/2)/1 -> Mux1/1
  Cos(Euler/2)/1 -> Mux1/2
  Mux1/1 -> e2/1, e3/1, e1/1, e0/1
  e0/1 -> Mux2/1
  e1/1 -> Mux2/2
  e2/1 -> Mux2/3
  e3/1 -> Mux2/4
  Euler angles/1 -> 1/2/1
  Mux2/1 -> Quaternions/1

== matlab function GTM_T2/MAG3 IMU/Embedded MATLAB Function ==
  data: omega input inherited; omega_dot input inherited; cg_pos input inherited; nbody input inherited; n_body output inherited; MAG3_pos parameter inherited
function n_body = accel_model(omega,omega_dot,cg_pos,nbody,MAG3_pos)
% Compute off-CG accelerometer corrections.  
% Inputs:
%       omega: body-axis angular rates, [p q r], in rad/sec

%   omega_dot: body-axis angular accelerations, [pdot qdot rdot], rad/sec^2
%       nbody: body-axis accels at CG [Nx Ny Nz], g
%      cg_pos: cg position, feet
%   MAG3_pos: accelerometer position, feet
%
% Note: cg and accel position must be in the same reference frame
%
% Author: Austin Murch (Austin.M.Murch@nasa.gov)
% Created: 11-2-2007

g0    = 32.174;

cg2accel = MAG3_pos' - cg_pos;

n_body =  nbody + (cross(omega,cross(omega,cg2accel)) + cross(omega_dot,cg2accel))/g0;

== matlab function GTM_T2/MIDG II 50 Hz/ENU to ECEF ==
  data: u input inherited; y output inherited
function y = fcn(u)
% Convert ENU position/velocity to ECEF, output both.

y = zeros(1,12); % initialize output length
 
d2r = pi/180; 
Vn  = u(1);
Ve  = u(2);
Vu  = u(3);
lat = u(4)*d2r;
lon = u(5)*d2r;
alt = u(6);

a2 = 4.068063159076900e+013; %m^2, Earth ellipsoid major axis squared
b2 = 4.040829998408706e+013; %m^2, Earth ellipsoid minor axis squared

N = a2/sqrt(a2*cos(lat)^2 + b2*sin(lat)^2);

XE = (alt + N)*cos(lat)*cos(lon);
YE = (alt + N)*cos(lat)*sin(lon);
ZE = (alt + N)*b2/a2*sin(lat);

VXE = Ve*sin(lat)*cos(lat) - Vn*sin(lon) - Vu*sin(lat)*cos(lon);
VYE = Ve*cos(lat)*sin(lon) + Vn*cos(lon) - Vu*sin(lat)*sin(lon);
VZE = Ve*sin(lat) + Vu*cos(lat);


y = [lat/d2r lon/d2r alt Vn Ve Vu XE YE ZE VXE VYE VZE];

== matlab function GTM_T2/MIDG II 50 Hz/Embedded MATLAB Function ==
  data: omega input inherited; omega_dot input inherited; cg_pos input inherited; nbody input inherited; n_body output inherited; MIDG_pos parameter inherited
function n_body = accel_model(omega,omega_dot,cg_pos,nbody,MIDG_pos)
% Compute off-CG accelerometer corrections.  
% Inputs:
%       omega: body-axis angular rates, [p q r], in rad/sec

%   omega_dot: body-axis angular accelerations, [pdot qdot rdot], rad/sec^2
%       nbody: body-axis accels at CG [Nx Ny Nz], g
%      cg_pos: cg position, feet
%    MIDG_pos: accelerometer position, feet
%
% Note: cg and accel position must be in the same reference frame
%
% Author: Austin Murch (Austin.M.Murch@nasa.gov)
% Created: 11-2-2007

g0    = 32.174;

cg2accel = MIDG_pos' - cg_pos;

n_body =  nbody + (cross(omega,cross(omega,cg2accel)) + cross(omega_dot,cg2accel))/g0;
